simulink model "gain_scheduling_sm_3_stateflow_WP5_seno_frequenza_1"  (R2023b)
settings: Solver=VariableStepAuto  StartTime=0.0  StopTime=10  RelTol=1e-3
values from neighbouring files (symbols this model uses):
  k1_sigma = [k1_sigma,double(subs(gains.k1, 'sigma', i))]    [gain_sheduling_WP5.m]
  k2_sigma = [k2_sigma,double(subs(gains.k2, 'sigma', i))]    [gain_sheduling_WP5.m]
settings Model: Creator=miche  LastModifiedBy=miche

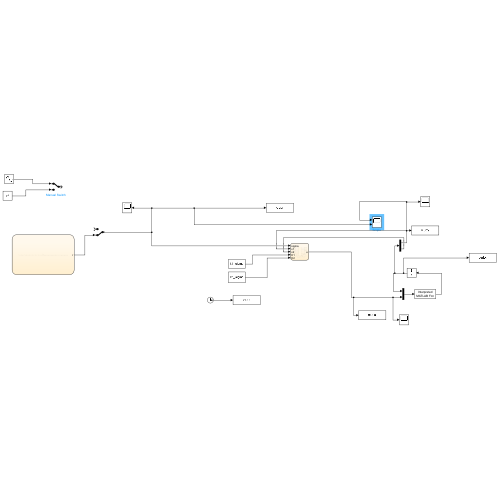
[thumbnail: Simulink's stored preview of the top-level diagram]
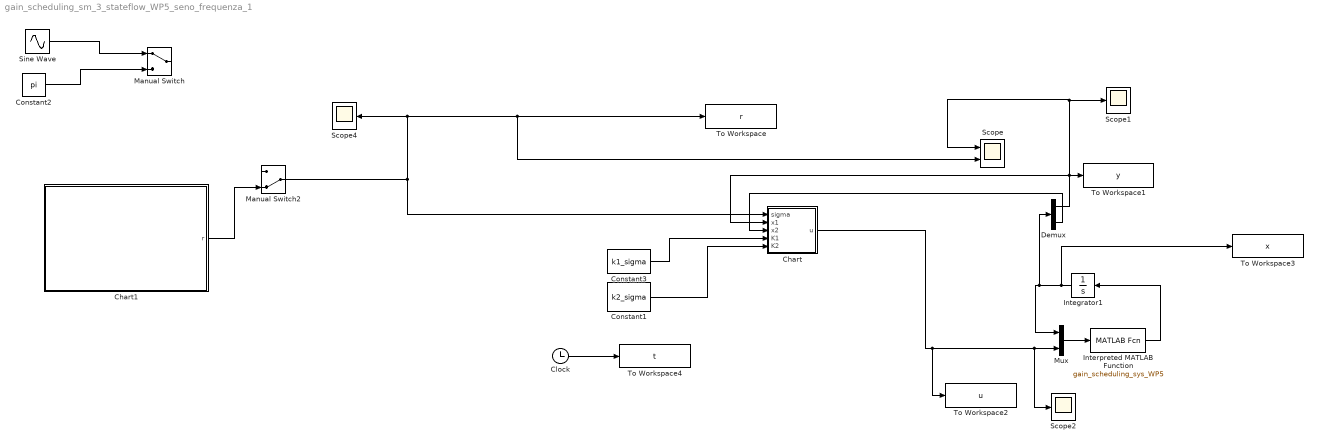
== system gain_scheduling_sm_3_stateflow_WP5_seno_frequenza_1 ==
  Chart : Stateflow chart  TreatAsAtomicUnit=on
  Chart1 : Stateflow chart  TreatAsAtomicUnit=on
  Clock : Clock
  Constant1 : Constant  Value=k2_sigma
  Constant2 : Constant  Value=pi
  Constant3 : Constant  Value=k1_sigma
  Demux : Demux  Outputs=2
  Integrator1 : Integrator
  Interpreted MATLAB Function : MATLABFcn  MATLABFcn=gain_scheduling_sys_WP5  OutputDimensions=2
  Manual Switch : ManualSwitch
  Manual Switch2 : ManualSwitch  CurrentSetting=0
  Mux : Mux  Inputs=2
  Scope : Scope  NumInputPorts=2
  Scope1 : Scope
  Scope2 : Scope
  Scope4 : Scope
  Sine Wave : Sin  SampleTime=0
  To Workspace : ToWorkspace  VariableName=r  SampleTime=-1
  To Workspace1 : ToWorkspace  VariableName=y  SampleTime=-1
  To Workspace2 : ToWorkspace  VariableName=u  SampleTime=-1
  To Workspace3 : ToWorkspace  VariableName=x  SampleTime=-1
  To Workspace4 : ToWorkspace  VariableName=t  SampleTime=-1
  wires:
  Sine Wave/1 -> Manual Switch/1
  Constant2/1 -> Manual Switch/2
  Constant1/1 -> Chart/5(K2)
  Constant3/1 -> Chart/4(K1)
  Clock/1 -> To Workspace4/1
  Chart1/1(r) -> Manual Switch2/2
  Manual Switch2/1 -> Scope/2, To Workspace/1, Scope4/1, Chart/1(sigma)
  Mux/1 -> Interpreted MATLAB Function/1
  Integrator1/1 -> To Workspace3/1, Demux/1, Mux/1
  Interpreted MATLAB Function/1 -> Integrator1/1
  Demux/1 -> Chart/2(x1), Scope/1, Scope1/1, To Workspace1/1
  Demux/2 -> Chart/3(x2)
  Chart/1(u) -> To Workspace2/1, Scope2/1, Mux/2

== stateflow chart gain_scheduling_sm_3_stateflow_WP5_seno_frequenza_1/Chart1 ==
  settings: updateMethod=DISCRETE  sampleTime=1e-3
  state S0
    d = 1;
  state S33
    r=-3.1416;
    d=1;
  state S35
    r=-2.9452;
  state S34
    r=-2.7489 ;
  state S26
    r=-2.5525 ;
  state S27
    r=-2.3562;
  state S25
    r=-2.1598;
  state S24
    r=-1.9635 ;
  state S21
    r=-1.7671 ;
  state S23
    r=-1.5708;
  state S22
    r=-1.3744 ;
  state S13
    r=-1.1781;
  state S14
    r=-0.9817 ;
  state S10
    r=-0.7854 ;
  state S12
    r=-0.5890;
  state S11
    r=-0.3927 ;
  state S4
    r=-0.1963;
  state S1
    r=0;
  state S2
    r=0.1963;
  state S3
    r=0.3927 ;
  state S6
    r=0.5890 ;
  state S8
    r=0.7854;
  state S9
    r=0.9817 ;
  state S7
    r=1.1781;
  state S19
    r=1.3744;
  state S20
    r=1.5708 ;
  state S15
    r=1.7671 ;
  state S17
    r=1.9635;
  state S16
    r=2.1598 ;
  state S18
    r=2.3562;
  state S28
    r=2.5525;
  state S30
    r=2.7489;
  state S29
    r=2.9452 ;
  state S31
    r=3.1416;
    d=0;
  (default) -> S0
  S0 -> S1
  S35 -> S34 [order 1] : [after(0.09817477042,sec) && d == 1]
  S25 -> S24 [order 1] : [after(0.09817477042,sec) && d == 1]
  S23 -> S22 [order 1] : [after(0.09817477042,sec) && d == 1]
  S13 -> S14 [order 1] : [after(0.09817477042,sec) && d == 1]
  S12 -> S11 [order 1] : [after(0.09817477042,sec) && d == 1]
  S1 -> S2 [order 1] : [after(0.09817477042, sec) && d == 1]
  S2 -> S3 [order 1] : [after(0.09817477042,sec) && d == 1]
  S8 -> S9 [order 1] : [after(0.09817477042,sec) && d == 1]
  S19 -> S20 [order 1] : [after(0.09817477042,sec) && d == 1]
  S17 -> S16 [order 1] : [after(0.09817477042,sec) && d == 1]
  S30 -> S29 [order 1] : [after(0.09817477042,sec) && d == 1]
  S33 -> S35 : [after(0.09817477042,sec) && d == 1]
  S21 -> S23 [order 2] : [after(0.09817477042,sec) && d == 1]
  S10 -> S12 [order 2] : [after(0.09817477042,sec) && d == 1]
  S4 -> S1 [order 1] : [after(0.09817477042,sec) && d == 1]
  S11 -> S4 [order 1] : [after(0.09817477042,sec) && d == 1]
  S27 -> S25 [order 2] : [after(0.09817477042,sec) && d == 1]
  S22 -> S13 [order 1] : [after(0.09817477042,sec) && d == 1]
  S6 -> S8 [order 2] : [after(0.09817477042,sec) && d == 1]
  S15 -> S17 [order 2] : [after(0.09817477042,sec) && d == 1]
  S28 -> S30 [order 1] : [after(0.09817477042,sec) && d == 1]
  S26 -> S27 [order 1] : [after(0.09817477042,sec) && d == 1]
  S24 -> S21 [order 1] : [after(0.09817477042,sec) && d == 1]
  S14 -> S10 [order 1] : [after(0.09817477042,sec) && d == 1]
  S34 -> S26 [order 1] : [after(0.09817477042,sec) && d == 1]
  S3 -> S6 [order 1] : [after(0.09817477042,sec) && d == 1]
  S9 -> S7 [order 1] : [after(0.09817477042,sec) && d == 1]
  S20 -> S15 [order 1] : [after(0.09817477042,sec) && d == 1]
  S16 -> S18 [order 1] : [after(0.09817477042,sec) && d == 1]
  S29 -> S31 [order 1] : [after(0.09817477042,sec) && d == 1]
  S7 -> S19 [order 2] : [after(0.09817477042,sec) && d == 1]
  S18 -> S28 [order 2] : [after(0.09817477042,sec) && d == 1]
  S4 -> S11 [order 2] : [after(0.09817477042,sec) && d == 0]
  S27 -> S26 [order 1] : [after(0.09817477042,sec) && d == 0]
  S21 -> S24 [order 1] : [after(0.09817477042,sec) && d == 0]
  S10 -> S14 [order 1] : [after(0.09817477042,sec) && d == 0]
  S34 -> S35 [order 2] : [after(0.09817477042,sec) && d == 0]
  S24 -> S25 [order 2] : [after(0.09817477042,sec) && d == 0]
  S22 -> S23 [order 2] : [after(0.09817477042,sec) && d == 0]
  S14 -> S13 [order 2] : [after(0.09817477042,sec) && d == 0]
  S11 -> S12 [order 2] : [after(0.09817477042,sec) && d == 0]
  S28 -> S18 [order 2] : [after(0.09817477042,sec) && d == 0]
  S26 -> S34 [order 2] : [after(0.09817477042,sec) && d == 0]
  S13 -> S22 [order 2] : [after(0.09817477042,sec) && d == 0]
  S35 -> S33 [order 2] : [after(0.09817477042,sec) && d == 0]
  S23 -> S21 [order 2] : [after(0.09817477042,sec) && d == 0]
  S12 -> S10 [order 2] : [after(0.09817477042,sec) && d == 0]
  S25 -> S27 [order 2] : [after(0.09817477042,sec) && d == 0]
  S7 -> S9 [order 1] : [after(0.09817477042,sec) && d == 0]
  S15 -> S20 [order 1] : [after(0.09817477042,sec) && d == 0]
  S18 -> S16 [order 1] : [after(0.09817477042,sec) && d == 0]
  S31 -> S29 : [after(0.09817477042,sec) && d == 0]
  S6 -> S3 [order 1] : [after(0.09817477042,sec) && d == 0]
  S1 -> S4 [order 2] : [after(0.09817477042,sec) && d == 0]
  S3 -> S2 [order 2] : [after(0.09817477042,sec) && d == 0]
  S9 -> S8 [order 2] : [after(0.09817477042,sec) && d == 0]
  S20 -> S19 [order 2] : [after(0.09817477042,sec) && d == 0]
  S16 -> S17 [order 2] : [after(0.09817477042,sec) && d == 0]
  S29 -> S30 [order 2] : [after(0.09817477042,sec) && d == 0]
  S8 -> S6 [order 2] : [after(0.09817477042,sec) && d == 0]
  S17 -> S15 [order 2] : [after(0.09817477042,sec) && d == 0]
  S30 -> S28 [order 2] : [after(0.09817477042,sec) && d == 0]
  S19 -> S7 [order 2] : [after(0.09817477042,sec) && d == 0]
  S2 -> S1 [order 2] : [after(0.09817477042,sec) && d == 0]
  data: r output; d local

== stateflow chart gain_scheduling_sm_3_stateflow_WP5_seno_frequenza_1/Chart ==
  settings: updateMethod=DISCRETE  sampleTime=1e-3
  state PI_controller_31
    during:
    u = -K1(31) * x1 - K2(31) * x2 + K1(31) * sigma;
  state Gain_Scheduler
  state PI_controller_0
    during:
    u = -K1(1) * x1 - K2(1) * x2 + K1(1) * sigma;
  state PI_controller_30
    during:
    u = -K1(30) * x1 - K2(30) * x2 + K1(30) * sigma;
  state PI_controller_1
    during:
    u = -K1(2) * x1 - K2(2) * x2 + K1(2) * sigma;
  state PI_controller_29
    during:
    u = -K1(29) * x1 - K2(29) * x2 + K1(29) * sigma;
  state PI_controller_2
    during:
    u = -K1(3) * x1 - K2(3) * x2 + K1(3) * sigma;
  state PI_controller_28
    during:
    u = -K1(28) * x1 - K2(28) * x2 + K1(28) * sigma;
  state PI_controller_3
    during:
    u = -K1(4) * x1 - K2(4) * x2 + K1(4) * sigma;
  state PI_controller_27
    during:
    u = -K1(27) * x1 - K2(27) * x2 + K1(27) * sigma;
  state PI_controller_4
    during:
    u = -K1(5) * x1 - K2(5) * x2 + K1(5) * sigma;
  state PI_controller_26
    during:
    u = -K1(26) * x1 - K2(26) * x2 + K1(26) * sigma;
  state PI_controller_5
    during:
    u = -K1(6) * x1 - K2(6) * x2 + K1(6) * sigma;
  state PI_controller_25
    during:
    u = -K1(25) * x1 - K2(25) * x2 + K1(25) * sigma;
  state PI_controller_6
    during:
    u = -K1(7) * x1 - K2(7) * x2 + K1(7) * sigma;
  state PI_controller_24
    during:
    u = -K1(24) * x1 - K2(24) * x2 + K1(24) * sigma;
  state PI_controller_7
    during:
    u = -K1(8) * x1 - K2(8) * x2 + K1(8) * sigma;
  state PI_controller_23
    during:
    u = -K1(24) * x1 - K2(24) * x2 + K1(24) * sigma;
  state PI_controller_8
    during:
    u = -K1(9) * x1 - K2(9) * x2 + K1(9) * sigma;
  state PI_controller_22
    during:
    u = -K1(23) * x1 - K2(23) * x2 + K1(23) * sigma;
  state PI_controller_9
    during:
    u = -K1(10) * x1 - K2(10) * x2 + K1(10) * sigma;
  state PI_controller_21
    during:
    u = -K1(22) * x1 - K2(22) * x2 + K1(22) * sigma;
  state PI_controller_10
    during:
    u = -K1(11) * x1 - K2(11) * x2 + K1(11) * sigma;
  state PI_controller_20
    during:
    u = -K1(21) * x1 - K2(21) * x2 + K1(21) * sigma;
  state PI_controller_11
    during:
    u = -K1(12) * x1 - K2(12) * x2 + K1(12) * sigma;
  state PI_controller_19
    during:
    u = -K1(20) * x1 - K2(20) * x2 + K1(20) * sigma;
  state PI_controller_12
    during:
    u = -K1(13) * x1 - K2(13) * x2 + K1(13) * sigma;
  state PI_controller_13
    during:
    u = -K1(14) * x1 - K2(14) * x2 + K1(14) * sigma;
  state PI_controller_18
    during:
    u = -K1(19) * x1 - K2(19) * x2 + K1(19) * sigma;
  state PI_controller_17
    during:
    u = -K1(18) * x1 - K2(18) * x2 + K1(18) * sigma;
  state PI_controller_14
    during:
    u = -K1(15) * x1 - K2(15) * x2 + K1(15) * sigma;
  state PI_controller_15
    during:
    u = -K1(16) * x1 - K2(16) * x2 + K1(16) * sigma;
  state PI_controller_16
    during:
    u = -K1(17) * x1 - K2(17) * x2 + K1(17) * sigma;
  PI_controller_31 -> Gain_Scheduler : [sigma~=3.1416]
  Gain_Scheduler -> PI_controller_31 [order 32] : [sigma==3.1416]
  (default) -> Gain_Scheduler
  PI_controller_30 -> Gain_Scheduler : [sigma~= 2.9452 ]
  PI_controller_0 -> Gain_Scheduler : [sigma~=-2.9452]
  Gain_Scheduler -> PI_controller_30 [order 31] : [sigma== 2.9452 ]
  Gain_Scheduler -> PI_controller_0 [order 1] : [sigma== -2.9452 ]
  PI_controller_29 -> Gain_Scheduler : [sigma~=2.7489]
  Gain_Scheduler -> PI_controller_1 [order 2] : [sigma==-2.7489]
  PI_controller_1 -> Gain_Scheduler : [sigma~=-2.7489]
  Gain_Scheduler -> PI_controller_29 [order 30] : [sigma==2.7489]
  PI_controller_28 -> Gain_Scheduler : [sigma~=2.5525]
  Gain_Scheduler -> PI_controller_2 [order 3] : [sigma==-2.5525]
  Gain_Scheduler -> PI_controller_28 [order 29] : [sigma==2.5525]
  PI_controller_2 -> Gain_Scheduler : [sigma~=-2.5525]
  PI_controller_27 -> Gain_Scheduler : [sigma~=2.3562]
  Gain_Scheduler -> PI_controller_3 [order 4] : [sigma==-2.3562]
  PI_controller_3 -> Gain_Scheduler : [sigma~=-2.3562]
  Gain_Scheduler -> PI_controller_27 [order 28] : [sigma==2.3562]
  PI_controller_26 -> Gain_Scheduler : [sigma~=2.1598]
  Gain_Scheduler -> PI_controller_4 [order 5] : [sigma==-2.1598]
  PI_controller_4 -> Gain_Scheduler : [sigma~=-2.1598]
  Gain_Scheduler -> PI_controller_26 [order 27] : [sigma==2.1598]
  PI_controller_25 -> Gain_Scheduler : [sigma~=1.9635]
  Gain_Scheduler -> PI_controller_5 [order 6] : [sigma==-1.9635]
  PI_controller_5 -> Gain_Scheduler : [sigma~=-1.9635]
  Gain_Scheduler -> PI_controller_25 [order 26] : [sigma==1.9635]
  Gain_Scheduler -> PI_controller_6 [order 7] : [sigma==-1.7671]
  PI_controller_24 -> Gain_Scheduler : [sigma~=1.7671]
  PI_controller_6 -> Gain_Scheduler : [sigma~=-1.7671]
  Gain_Scheduler -> PI_controller_24 [order 25] : [sigma==1.7671]
  Gain_Scheduler -> PI_controller_7 [order 8] : [sigma==-1.5708]
  PI_controller_23 -> Gain_Scheduler : [sigma~=1.5708]
  PI_controller_7 -> Gain_Scheduler : [sigma~=-1.5708]
  Gain_Scheduler -> PI_controller_23 [order 24] : [sigma==1.5708]
  PI_controller_22 -> Gain_Scheduler : [sigma~=1.3744 ]
  Gain_Scheduler -> PI_controller_8 [order 9] : [sigma==-1.3744 ]
  Gain_Scheduler -> PI_controller_22 [order 23] : [sigma==1.3744 ]
  PI_controller_8 -> Gain_Scheduler : [sigma~=-1.3744 ]
  PI_controller_21 -> Gain_Scheduler : [sigma~=1.1781]
  Gain_Scheduler -> PI_controller_21 [order 22] : [sigma==1.1781]
  Gain_Scheduler -> PI_controller_9 [order 10] : [sigma==-1.1781]
  PI_controller_9 -> Gain_Scheduler : [sigma~=-1.1781]
  PI_controller_20 -> Gain_Scheduler : [sigma~=0.9817]
  Gain_Scheduler -> PI_controller_10 [order 11] : [sigma==-0.9817]
  Gain_Scheduler -> PI_controller_20 [order 21] : [sigma==0.9817]
  PI_controller_10 -> Gain_Scheduler : [sigma~=-0.9817]
  Gain_Scheduler -> PI_controller_19 [order 20] : [sigma==0.7854]
  PI_controller_19 -> Gain_Scheduler : [sigma~=0.7854]
  PI_controller_11 -> Gain_Scheduler : [sigma~=-0.7854]
  Gain_Scheduler -> PI_controller_11 [order 12] : [sigma==-0.7854]
  PI_controller_18 -> Gain_Scheduler : [sigma~= 0.5890]
  PI_controller_14 -> Gain_Scheduler : [sigma~=-0.1963]
  Gain_Scheduler -> PI_controller_14 [order 15] : [sigma==-0.1963]
  Gain_Scheduler -> PI_controller_18 [order 19] : [sigma== 0.5890]
  Gain_Scheduler -> PI_controller_17 [order 18] : [sigma==0.3927 ]
  PI_controller_17 -> Gain_Scheduler : [sigma~=0.3927 ]
  PI_controller_16 -> Gain_Scheduler : [sigma~= 0.1963]
  Gain_Scheduler -> PI_controller_16 [order 17] : [sigma== 0.1963]
  Gain_Scheduler -> PI_controller_15 [order 16] : [sigma== 0]
  PI_controller_15 -> Gain_Scheduler : [sigma~= 0]
  PI_controller_13 -> Gain_Scheduler : [sigma~=-0.3927 ]
  Gain_Scheduler -> PI_controller_13 [order 14] : [sigma==-0.3927 ]
  PI_controller_12 -> Gain_Scheduler : [sigma~= -0.5890]
  Gain_Scheduler -> PI_controller_12 [order 13] : [sigma== -0.5890]
  data: sigma input; x1 input; x2 input; K1 input; K2 input; u output
